simulink model "FinalModel"  (R2022a)
settings: Solver=VariableStepAuto  StartTime=0.0  StopTime=1  RelTol=1e-3
model workspace (MAT data in the model file):
  a = 50
  x = 100
undefined symbols (not defined in the file): gray
libraries: visionsources x2
settings Model: Creator=Dell  LastModifiedBy=Dell
settings ConfigComp: CovEnable=on  CovScope=ReferencedModels  RecordCoverage=on  CovForceBlockReductionOff=off  CovEnableCumulative=off

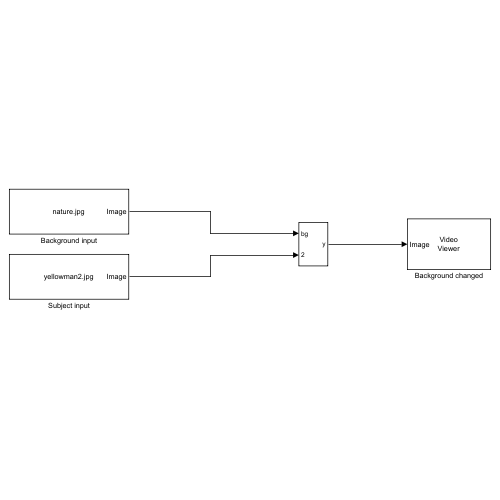
[thumbnail: Simulink's stored preview of the top-level diagram]
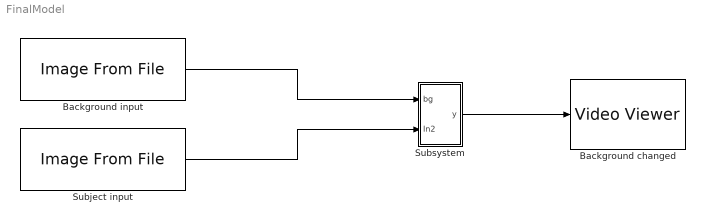
== system FinalModel ==
  Background changed : VideoViewer  colormapValue=gray(256)  FigPos=[1 862 1536 764]
  Background input : visionsources/Image From File  Tag=vipblks_nd  FileName=F:\LTTS\project\nature.jpg  Ts=inf  imagePorts=One multidimensional signal  OutPortLabels=R|G|B  ImageDataType=Inherit from input image  sdImageDataType=uint(8)  Signed=on  WordLength=16  FractionLengthMode=User-defined  FractionLength=15
  Subject input : visionsources/Image From File  Tag=vipblks_nd  FileName=F:\LTTS\project\yellowman2.jpg  Ts=inf  imagePorts=One multidimensional signal  OutPortLabels=R|G|B  ImageDataType=Inherit from input image  sdImageDataType=uint(8)  Signed=on  WordLength=16  FractionLengthMode=User-defined  FractionLength=15
  Subsystem : Subsystem
  wires:
  Background input/1 -> Subsystem/1(bg)
  Subject input/1 -> Subsystem/2(In2)
  Subsystem/1(y) -> Background changed/1

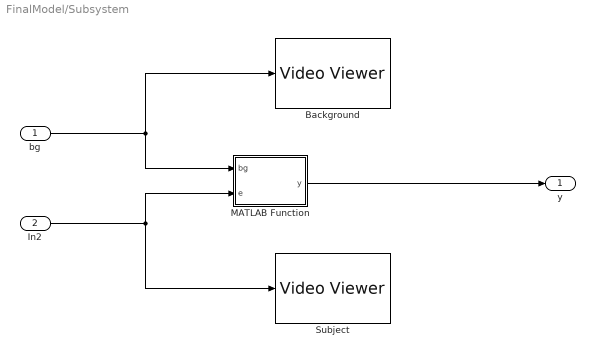
== system FinalModel/Subsystem ==
  bg : Inport
  In2 : Inport  Port=2
  Background : VideoViewer  FigPos=[1 862 1536 764]
  MATLAB Function : MATLAB Function  TreatAsAtomicUnit=on
  Subject : VideoViewer  colormapValue=gray(256)  FigPos=[1 862 1536 764]
  y : Outport
  wires:
  In2/1 -> MATLAB Function/2(e), Subject/1
  bg/1 -> Background/1, MATLAB Function/1(bg)
  MATLAB Function/1(y) -> y/1

== matlab function FinalModel/Subsystem/MATLAB Function ==
  data: bg input; y output; e input
function y = fcn(bg, e)



function [BW,maskedRGBImage] = createMask(RGB)

% Convert RGB image to chosen color space
I = rgb2hsv(RGB);

% Define thresholds for channel 1 based on histogram settings
channel1Min = 0.196;
channel1Max = 0.000;

% Define thresholds for channel 2 based on histogram settings
channel2Min = 0.000;
channel2Max = 0.236;

% Define thresholds for channel 3 based on histogram settings
channel3Min = 0.322;
channel3Max = 1.000;

% Create mask based on chosen histogram thresholds
sliderBW = ( (I(:,:,1) >= channel1Min) | (I(:,:,1) <= channel1Max) ) & ...
    (I(:,:,2) >= channel2Min ) & (I(:,:,2) <= channel2Max) & ...
    (I(:,:,3) >= channel3Min ) & (I(:,:,3) <= channel3Max);
BW = sliderBW;

% Invert mask
BW = ~BW;

% Initialize output masked image based on input image.
maskedRGBImage = RGB;

% Set background pixels where BW is false to zero.
maskedRGBImage(repmat(~BW,[1 1 3])) = 0;

end

[r c b]=size(e);
gm=imresize(bg,[r c]);
mkdir=createMask(e);
gs=gm.*uint8(~mkdir);

gm=bg;
y=(gs+e.*uint8(mkdir));
end
